simulink model "newthing"  (Simulink 9.1)
settings: Solver=FixedStepAuto  StartTime=0.0  StopTime=tT  FixedStep=dt  RelTol=1e-4  EnableMultiTasking=on
values from neighbouring files (symbols this model uses):
  A = LinearAnalysisToolProject.LocalVariables(2).Value.A    [KalmanFiltBoi.m]    (also in newthingtest.m; newthingtest2.m)
  a1 = 16.235    [LoadQuadrotorConst_XPro1a.m]
  a2 = 17.912    [LoadQuadrotorConst_XPro1a.m]
  a3 = 17.914    [LoadQuadrotorConst_XPro1a.m]
  a4 = 18.161    [LoadQuadrotorConst_XPro1a.m]
  B = LinearAnalysisToolProject.LocalVariables(2).Value.B    [KalmanFiltBoi.m]    (also in newthingtest.m; newthingtest2.m)
  b1 = -0.5036    [LoadQuadrotorConst_XPro1a.m]
  b2 = -12.728    [LoadQuadrotorConst_XPro1a.m]
  b3 = -6.5646    [LoadQuadrotorConst_XPro1a.m]
  b4 = -7.4637    [LoadQuadrotorConst_XPro1a.m]
  c = 0.0002    [LoadQuadrotorConst_XPro1a.m]
  c_mi_x = 170    [LoadQuadrotorConst_XPro1a.m]
  c_mi_y = 170    [LoadQuadrotorConst_XPro1a.m]
  c_mi_z = 40    [LoadQuadrotorConst_XPro1a.m]
  Cc = LinearAnalysisToolProject.LocalVariables(2).Value.C    [newthingtest2.m]
  co_x = 1.7    [LoadQuadrotorConst_XPro1a.m]
  co_y = 1.7    [LoadQuadrotorConst_XPro1a.m]
  co_z = 90.7    [LoadQuadrotorConst_XPro1a.m]
  d = 0.0071    [LoadQuadrotorConst_XPro1a.m]
  d_omega_R10 = 9.1275    [initial_conditions.m]
  d_omega_R20 = 8.955    [initial_conditions.m]
  d_omega_R30 = 8.61    [initial_conditions.m]
  d_omega_R40 = 8.543    [initial_conditions.m]
  dfi_0 = 0    [initial_conditions.m]
  dpsi_0 = 0    [initial_conditions.m]
  dt = 1    [cvx_guidance.m]    (also in newthingtest2.m = 0.01; test_cvx.m = 0.05)
  dtheta_0 = 0    [initial_conditions.m]
  dx_0 = 0    [initial_conditions.m]
  dy_0 = 0    [initial_conditions.m]
  dz_0 = 0    [initial_conditions.m]
  f = 5e-6    (= 5e-06)    [LoadQuadrotorConst_XPro1a.m]
  fi_0 = 0    [initial_conditions.m]
  G = eye(16)    [newthingtest2.m]
  g = 0.0008    [LoadQuadrotorConst_XPro1a.m]    (also in cvx_guidance.m = 9.81)
  ga = 9.807    [LoadQuadrotorConst_XPro1a.m]
  H = eye(16)    [newthingtest2.m]
  h = -0.0282    [LoadQuadrotorConst_XPro1a.m]
  hover = [V1_WP;V2_WP;V3_WP;V4_WP]    [initial_conditions.m]
  Ixx = 2.1385*100    (= 213.85)    [LoadQuadrotorConst_XPro1a.m]
  Iyy = Ixx    (= 213.85)    [LoadQuadrotorConst_XPro1a.m]
  Izz = 3.7479*100    (= 374.79)    [LoadQuadrotorConst_XPro1a.m]
  Jr = 4.86851*0.1    (= 0.486851)    [LoadQuadrotorConst_XPro1a.m]
  K = C(1:4,:)    [newthingtest2.m]
  L = 0.422    [LoadQuadrotorConst_XPro1a.m]
  m = 2.1    [LoadQuadrotorConst_XPro1a.m]    (also in cvx_guidance.m; plot_all_data3D.m = exp(z))
  psi_0 = 0    [initial_conditions.m]
  S_0_0 = 10^7*eye(16)    [newthingtest2.m]
  stateref = [0 0 0 0 0 0 0 0 0 0 0 0 0 0 0 0]'    [newthingtest.m]    (also in newthingtest2.m = [35 0 35 0 50 0 0 0 0 0 0 0 0 0 0 0]')
  Sv = Sv^4    [newthingtest2.m]
  Sw = Sv    [newthingtest2.m]
  Tau = 0.1    [LoadQuadrotorConst_XPro1a.m]
  theta_0 = 0    [initial_conditions.m]
  x_0 = 0    [initial_conditions.m]
  x_0_0 = [x_0 dx_0 y_0 dy_0 z_0 dz_0      fi_0 dfi_0 theta_0 dtheta_0 psi_0 dpsi_0 hover.'].'    [initial_conditions.m]
  y_0 = 0    [initial_conditions.m]
  z_0 = 30    [initial_conditions.m]
settings Model: Creator=Jake  LastModifiedBy=Padraig Lysandrou
settings DataIOCC: LimitDataPoints=on  SignalLoggingSaveFormat=ModelDataLogs
settings OptimizationCC: InitFltsAndDblsToZero=on
settings DebuggingCC: SaveWithParameterizedLinksMsg=none  SignalResolutionControl=TryResolveAllWithWarning  SolverPrmCheckMsg=warning  MultiTaskDSMMsg=warning  MultiTaskCondExecSysMsg=none  FcnCallInpInsideContextMsg=warning
settings SFSimCC: SimParseCustomCode=off
settings GRTTargetCC: TargetFcnLib=ansi_tfl_tmw.mat

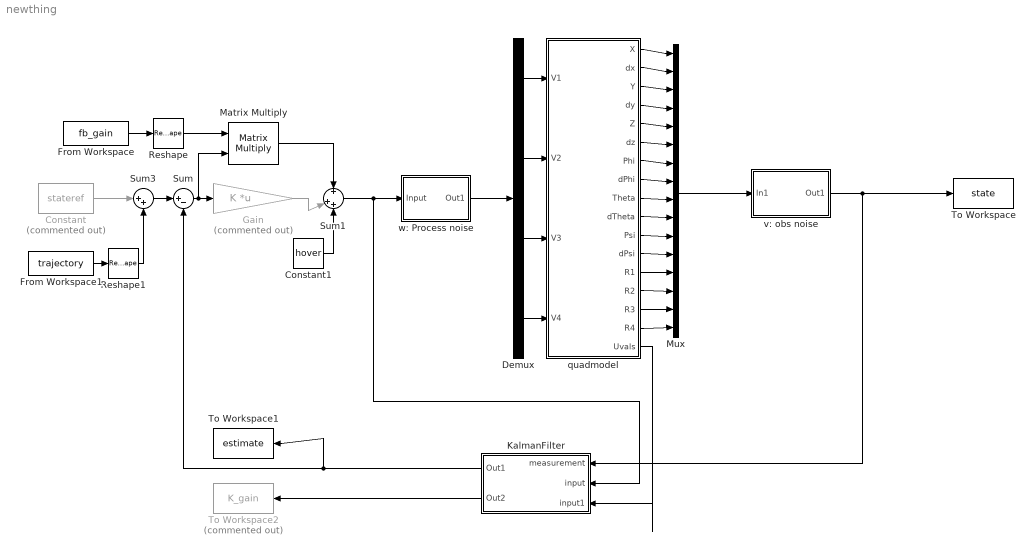
== system newthing ==
  Constant : Constant  Commented=on  Value=stateref
  Constant1 : Constant  Value=hover
  Demux : Demux
  From Workspace : FromWorkspace  VariableName=fb_gain  SampleTime=0
  From Workspace1 : FromWorkspace  VariableName=trajectory  SampleTime=0
  Gain : Gain  Commented=on  Gain=K  Multiplication=Matrix(K*u) (u vector)
  KalmanFilter : Subsystem
  Matrix Multiply : Product  Multiplication=Matrix(*)
  Mux : Mux  Inputs=16
  Reshape : Reshape  OutputDimensionality=Customize  OutputDimensions=[4,16]
  Reshape1 : Reshape  OutputDimensionality=Customize  OutputDimensions=[16,1]
  Sum : Sum  Inputs=|+-
  Sum1 : Sum  Inputs=+|++
  Sum3 : Sum  Inputs=|++
  To Workspace : ToWorkspace  VariableName=state  SaveFormat=Timeseries  SampleTime=-1
  To Workspace1 : ToWorkspace  VariableName=estimate  SaveFormat=Timeseries  SampleTime=-1
  To Workspace2 : ToWorkspace  Commented=on  VariableName=K_gain  SaveFormat=Timeseries  SampleTime=-1
  quadmodel : Subsystem
  v: obs noise : Subsystem
  w: Process noise : Subsystem
  wires:
  quadmodel/1(X) -> Mux/1
  quadmodel/2(dx) -> Mux/2
  quadmodel/3(Y) -> Mux/3
  quadmodel/4(dy) -> Mux/4
  quadmodel/5(Z) -> Mux/5
  quadmodel/6(dz) -> Mux/6
  quadmodel/7(Phi) -> Mux/7
  quadmodel/8(dPhi) -> Mux/8
  quadmodel/9(Theta) -> Mux/9
  quadmodel/10(dTheta) -> Mux/10
  quadmodel/11(Psi) -> Mux/11
  quadmodel/12(dPsi) -> Mux/12
  Demux/1 -> quadmodel/1(V1)
  Demux/2 -> quadmodel/2(V2)
  Demux/3 -> quadmodel/3(V3)
  Demux/4 -> quadmodel/4(V4)
  quadmodel/13(R1) -> Mux/13
  quadmodel/14(R2) -> Mux/14
  quadmodel/15(R3) -> Mux/15
  quadmodel/16(R4) -> Mux/16
  Constant1/1 -> Sum1/3
  From Workspace/1 -> Reshape/1
  Reshape/1 -> Matrix Multiply/1
  Sum/1 -> Matrix Multiply/2, Gain/1
  Matrix Multiply/1 -> Sum1/1
  Gain/1 -> Sum1/2
  From Workspace1/1 -> Reshape1/1
  Sum3/1 -> Sum/1
  Reshape1/1 -> Sum3/2
  Constant/1 -> Sum3/1
  Mux/1 -> v: obs noise/1(In1)
  Sum1/1 -> KalmanFilter/2(input), w: Process noise/1(Input)
  v: obs noise/1(Out1) -> KalmanFilter/1(measurement), To Workspace/1
  w: Process noise/1(Out1) -> Demux/1
  KalmanFilter/2(Out2) -> To Workspace2/1
  KalmanFilter/1(Out1) -> To Workspace1/1, Sum/2
  quadmodel/17(Uvals) -> KalmanFilter/3(input1)

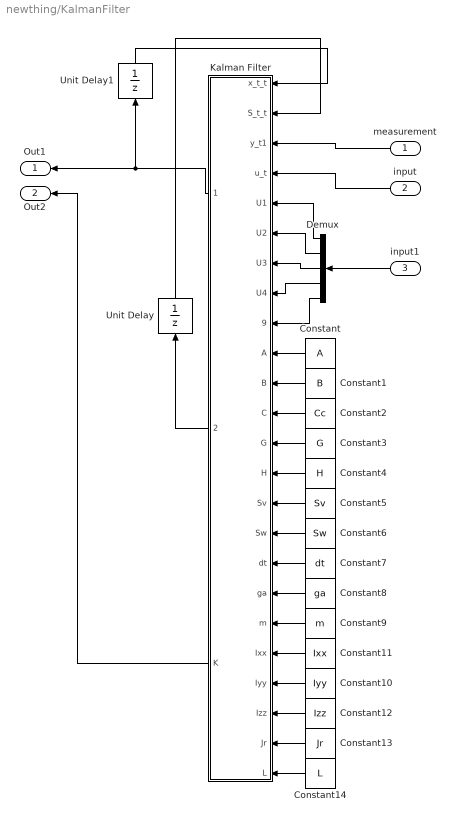
== system newthing/KalmanFilter ==
  measurement : Inport
  input : Inport  Port=2
  input1 : Inport  Port=3
  Constant : Constant  Value=A
  Constant1 : Constant  Value=B
  Constant10 : Constant  Value=Iyy
  Constant11 : Constant  Value=Ixx
  Constant12 : Constant  Value=Izz
  Constant13 : Constant  Value=Jr
  Constant14 : Constant  Value=L
  Constant2 : Constant  Value=Cc
  Constant3 : Constant  Value=G
  Constant4 : Constant  Value=H
  Constant5 : Constant  Value=Sv
  Constant6 : Constant  Value=Sw
  Constant7 : Constant  Value=dt
  Constant8 : Constant  Value=ga
  Constant9 : Constant  Value=m
  Demux : Demux  Outputs=5
  Kalman Filter : MATLAB Function  TreatAsAtomicUnit=on
  Unit Delay : UnitDelay  InitialCondition=S_0_0  SampleTime=-1
  Unit Delay1 : UnitDelay  InitialCondition=x_0_0  SampleTime=-1
  Out1 : Outport
  Out2 : Outport  Port=2
  wires:
  Kalman Filter/1(x_t1_t1) -> Unit Delay1/1, Out1/1
  Constant/1 -> Kalman Filter/10(A)
  Constant1/1 -> Kalman Filter/11(B)
  Constant2/1 -> Kalman Filter/12(C)
  Kalman Filter/2(S_t1_t1) -> Unit Delay/1
  Unit Delay/1 -> Kalman Filter/2(S_t_t)
  Unit Delay1/1 -> Kalman Filter/1(x_t_t)
  Constant3/1 -> Kalman Filter/13(G)
  Constant4/1 -> Kalman Filter/14(H)
  Constant5/1 -> Kalman Filter/15(Sv)
  Constant6/1 -> Kalman Filter/16(Sw)
  Kalman Filter/3(K) -> Out2/1
  measurement/1 -> Kalman Filter/3(y_t1)
  Demux/1 -> Kalman Filter/5(U1)
  Demux/2 -> Kalman Filter/6(U2)
  Demux/3 -> Kalman Filter/7(U3)
  Demux/4 -> Kalman Filter/8(U4)
  Demux/5 -> Kalman Filter/9(Omega)
  input1/1 -> Demux/1
  input/1 -> Kalman Filter/4(u_t)
  Constant7/1 -> Kalman Filter/17(dt)
  Constant8/1 -> Kalman Filter/18(ga)
  Constant9/1 -> Kalman Filter/19(m)
  Constant10/1 -> Kalman Filter/21(Iyy)
  Constant11/1 -> Kalman Filter/20(Ixx)
  Constant12/1 -> Kalman Filter/22(Izz)
  Constant14/1 -> Kalman Filter/24(L)
  Constant13/1 -> Kalman Filter/23(Jr)

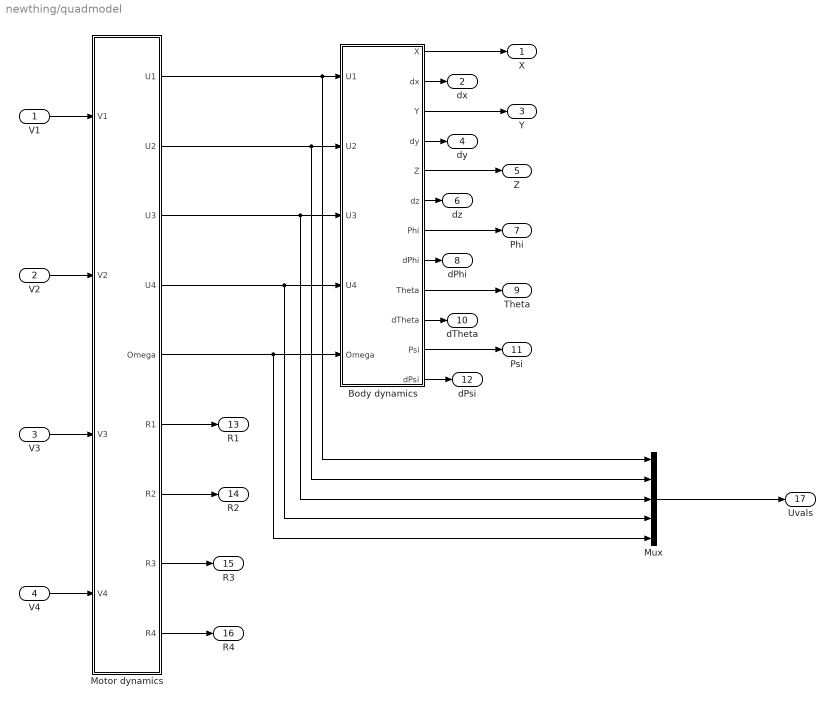
== system newthing/quadmodel ==
  V1 : Inport
  V2 : Inport  Port=2
  V3 : Inport  Port=3
  V4 : Inport  Port=4
  Body dynamics : Subsystem
  Motor dynamics : Subsystem
  Mux : Mux  Inputs=5
  X : Outport
  dx : Outport  Port=2
  Y : Outport  Port=3
  dy : Outport  Port=4
  Z : Outport  Port=5
  dz : Outport  Port=6
  Phi : Outport  Port=7
  dPhi : Outport  Port=8
  Theta : Outport  Port=9
  dTheta : Outport  Port=10
  Psi : Outport  Port=11
  dPsi : Outport  Port=12
  R1 : Outport  Port=13
  R2 : Outport  Port=14
  R3 : Outport  Port=15
  R4 : Outport  Port=16
  Uvals : Outport  Port=17
  wires:
  Motor dynamics/1(U1) -> Body dynamics/1(U1), Mux/1
  Motor dynamics/2(U2) -> Body dynamics/2(U2), Mux/2
  Motor dynamics/3(U3) -> Body dynamics/3(U3), Mux/3
  Motor dynamics/4(U4) -> Body dynamics/4(U4), Mux/4
  Motor dynamics/5(Omega) -> Body dynamics/5(Omega), Mux/5
  Body dynamics/7(Phi) -> Phi/1
  Body dynamics/9(Theta) -> Theta/1
  Body dynamics/11(Psi) -> Psi/1
  Body dynamics/1(X) -> X/1
  V1/1 -> Motor dynamics/1(V1)
  Body dynamics/3(Y) -> Y/1
  V2/1 -> Motor dynamics/2(V2)
  Body dynamics/5(Z) -> Z/1
  V3/1 -> Motor dynamics/3(V3)
  V4/1 -> Motor dynamics/4(V4)
  Body dynamics/2(dx) -> dx/1
  Body dynamics/4(dy) -> dy/1
  Body dynamics/6(dz) -> dz/1
  Body dynamics/8(dPhi) -> dPhi/1
  Body dynamics/10(dTheta) -> dTheta/1
  Body dynamics/12(dPsi) -> dPsi/1
  Motor dynamics/6(R1) -> R1/1
  Motor dynamics/7(R2) -> R2/1
  Motor dynamics/8(R3) -> R3/1
  Motor dynamics/9(R4) -> R4/1
  Mux/1 -> Uvals/1

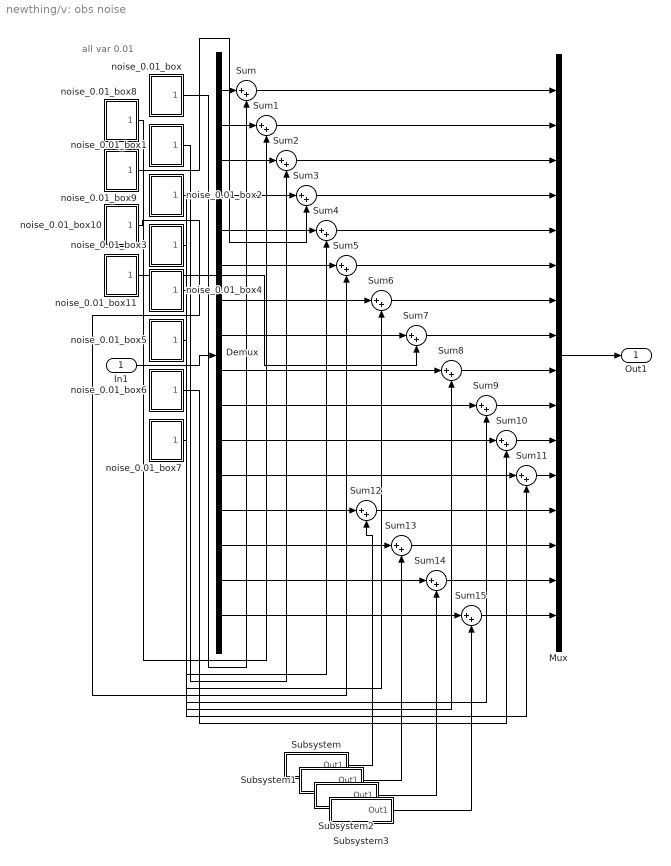
== system newthing/v: obs noise ==
  note: all var 0.01
  In1 : Inport
  Demux : Demux  Outputs=16
  Mux : Mux  Inputs=16
  Subsystem : Subsystem
  Subsystem1 : Subsystem
  Subsystem2 : Subsystem
  Subsystem3 : Subsystem
  Sum{,1..15} (16 alike) : Sum  Inputs=|++
  noise_0.01_box : Subsystem
  noise_0.01_box1 : Subsystem
  noise_0.01_box10 : Subsystem
  noise_0.01_box11 : Subsystem
  noise_0.01_box2 : Subsystem
  noise_0.01_box3 : Subsystem
  noise_0.01_box4 : Subsystem
  noise_0.01_box5 : Subsystem
  noise_0.01_box6 : Subsystem
  noise_0.01_box7 : Subsystem
  noise_0.01_box8 : Subsystem
  noise_0.01_box9 : Subsystem
  Out1 : Outport
  wires:
  Demux/2 -> Sum1/1
  Demux/1 -> Sum/1
  Sum2/1 -> Mux/3
  Sum/1 -> Mux/1
  Demux/3 -> Sum2/1
  Demux/4 -> Sum3/1
  Sum3/1 -> Mux/4
  Demux/5 -> Sum4/1
  Sum4/1 -> Mux/5
  Sum1/1 -> Mux/2
  Demux/6 -> Sum5/1
  Sum5/1 -> Mux/6
  Demux/7 -> Sum6/1
  Sum6/1 -> Mux/7
  Demux/8 -> Sum7/1
  Sum7/1 -> Mux/8
  Demux/9 -> Sum8/1
  Sum8/1 -> Mux/9
  Demux/10 -> Sum9/1
  Sum9/1 -> Mux/10
  Demux/11 -> Sum10/1
  Sum10/1 -> Mux/11
  Demux/12 -> Sum11/1
  Sum11/1 -> Mux/12
  In1/1 -> Demux/1
  Mux/1 -> Out1/1
  Demux/13 -> Sum12/1
  Sum12/1 -> Mux/13
  Demux/14 -> Sum13/1
  Sum13/1 -> Mux/14
  Demux/15 -> Sum14/1
  Sum14/1 -> Mux/15
  Demux/16 -> Sum15/1
  Sum15/1 -> Mux/16
  noise_0.01_box/1(Out1) -> Sum/2
  noise_0.01_box8/1(Out1) -> Sum1/2
  noise_0.01_box1/1(Out1) -> Sum2/2
  noise_0.01_box9/1(Out1) -> Sum3/2
  noise_0.01_box2/1(Out1) -> Sum4/2
  noise_0.01_box10/1(Out1) -> Sum5/2
  noise_0.01_box3/1(Out1) -> Sum6/2
  noise_0.01_box11/1(Out1) -> Sum7/2
  noise_0.01_box4/1(Out1) -> Sum8/2
  noise_0.01_box5/1(Out1) -> Sum9/2
  noise_0.01_box6/1(Out1) -> Sum10/2
  noise_0.01_box7/1(Out1) -> Sum11/2
  Subsystem/1(Out1) -> Sum12/2
  Subsystem1/1(Out1) -> Sum13/2
  Subsystem2/1(Out1) -> Sum14/2
  Subsystem3/1(Out1) -> Sum15/2

== system newthing/w: Process noise ==
  Input : Inport
  Demux : Demux
  Mux : Mux
  Subsystem : Subsystem
  Subsystem1 : Subsystem
  Subsystem2 : Subsystem
  Subsystem3 : Subsystem
  Sum{,1..3} (4 alike) : Sum  Inputs=|++
  Out1 : Outport
  wires:
  Input/1 -> Demux/1
  Demux/1 -> Sum/1
  Demux/2 -> Sum1/1
  Mux/1 -> Out1/1
  Sum/1 -> Mux/1
  Sum1/1 -> Mux/2
  Demux/3 -> Sum2/1
  Demux/4 -> Sum3/1
  Sum2/1 -> Mux/3
  Sum3/1 -> Mux/4
  Subsystem/1(Out1) -> Sum3/2
  Subsystem1/1(Out1) -> Sum2/2
  Subsystem2/1(Out1) -> Sum1/2
  Subsystem3/1(Out1) -> Sum/2

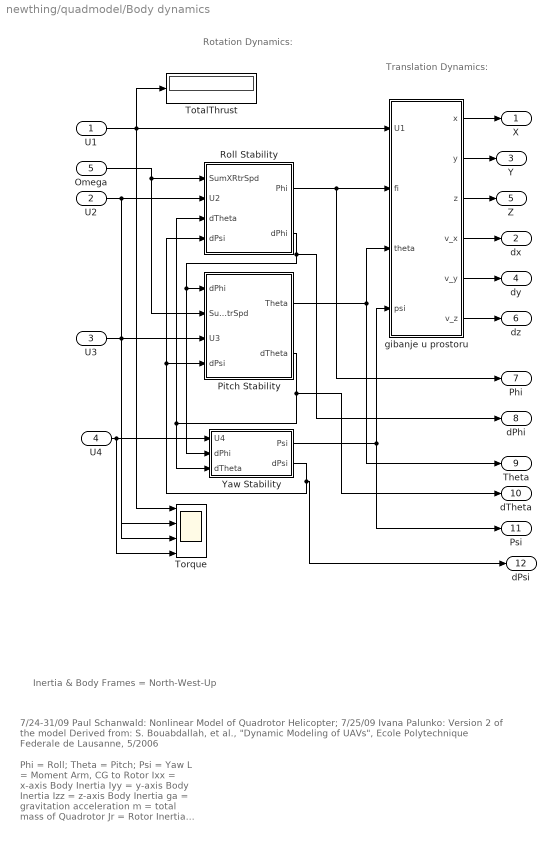
== system newthing/quadmodel/Body dynamics ==
  note: Inertia & Body Frames = North-West-Up
  note: Rotation
      | Dynamics:
  note: Translation
      | Dynamics:
  note: Phi = Roll; Theta = Pitch; Psi = Yaw
      | L = Moment Arm, CG to Rotor
      | Ixx = x-axis Body Inertia
      | Iyy = y-axis Body Inertia
      | Izz = z-axis Body Inertia
      | ga = gravitation acceleration
      | m = total mass of Quadrotor
      | Jr = Rotor Inertia
      | a,b = Volts-to-Rotor Speed Consts
      | c,d,e = RtrSpd-to-Thrust Fcn Consts
      | f,g,h = RtrSpd-to-Drag Fcn Consts
      | Tau = Motor Time Const
  note: 7/24-31/09  Paul Schanwald:  Nonlinear Model of Quadrotor Helicopter; 7/25/09 Ivana Palunko: Version 2 of the model
      | Derived from: S. Bouabdallah, et al., "Dynamic Modeling of UAVs", Ecole Polytechnique Federale de Lausanne, 5/2006
  U1 : Inport
  U2 : Inport  Port=2
  U3 : Inport  Port=3
  U4 : Inport  Port=4
  Omega : Inport  Port=5
  Pitch Stability : Subsystem
  Roll Stability : Subsystem
  Torque : Scope  NumInputPorts=4
  TotalThrust : Display
  Yaw Stability : Subsystem
  gibanje u prostoru : Subsystem
  X : Outport
  dx : Outport  Port=2
  Y : Outport  Port=3
  dy : Outport  Port=4
  Z : Outport  Port=5
  dz : Outport  Port=6
  Phi : Outport  Port=7
  dPhi : Outport  Port=8
  Theta : Outport  Port=9
  dTheta : Outport  Port=10
  Psi : Outport  Port=11
  dPsi : Outport  Port=12
  wires:
  U4/1 -> Yaw Stability/1(U4), Torque/4
  U3/1 -> Pitch Stability/3(U3), Torque/3
  U1/1 -> TotalThrust/1, gibanje u prostoru/1(U1), Torque/1
  gibanje u prostoru/3(z) -> Z/1
  gibanje u prostoru/2(y) -> Y/1
  gibanje u prostoru/1(x) -> X/1
  U2/1 -> Roll Stability/2(U2), Torque/2
  Omega/1 -> Roll Stability/1(SumXRtrSpd), Pitch Stability/2(SumYRtrSpd)
  Roll Stability/2(dPhi) -> dPhi/1, Pitch Stability/1(dPhi), Yaw Stability/2(dPhi)
  Pitch Stability/2(dTheta) -> dTheta/1, Yaw Stability/3(dTheta), Roll Stability/3(dTheta)
  Yaw Stability/2(dPsi) -> dPsi/1, Roll Stability/4(dPsi), Pitch Stability/4(dPsi)
  Roll Stability/1(Phi) -> gibanje u prostoru/2(fi), Phi/1
  Pitch Stability/1(Theta) -> gibanje u prostoru/3(theta), Theta/1
  Yaw Stability/1(Psi) -> Psi/1, gibanje u prostoru/4(psi)
  gibanje u prostoru/6(v_z) -> dz/1
  gibanje u prostoru/4(v_x) -> dx/1
  gibanje u prostoru/5(v_y) -> dy/1

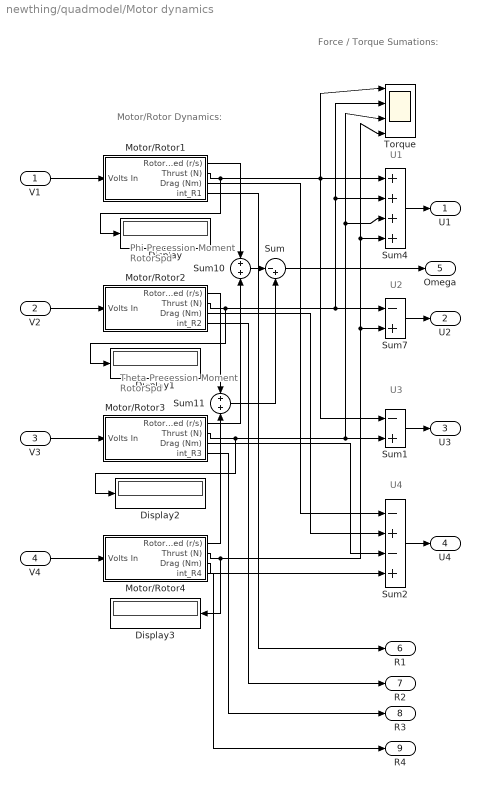
== system newthing/quadmodel/Motor dynamics ==
  note: Theta Precession
      | Moment RotorSpd
  note: Phi Precession
      | Moment RotorSpd
  note: Motor/Rotor
      | Dynamics:
  note: Force / Torque
      | Sumations:
  note: U4
  note: U3
  note: U2
  note: U1
  V1 : Inport
  V2 : Inport  Port=2
  V3 : Inport  Port=3
  V4 : Inport  Port=4
  Display{,1..3} (4 alike) : Display
  Motor/Rotor1 : Subsystem
  Motor/Rotor2 : Subsystem
  Motor/Rotor3 : Subsystem
  Motor/Rotor4 : Subsystem
  Sum : Sum  Inputs=|-+
  Sum1 : Sum  Inputs=-+
  Sum10 : Sum  Inputs=+|+
  Sum11 : Sum  Inputs=+|+
  Sum2 : Sum  Inputs=-+-+
  Sum4 : Sum  Inputs=++++
  Sum7 : Sum  Inputs=-+
  Torque : Scope  NumInputPorts=4
  U1 : Outport
  U2 : Outport  Port=2
  U3 : Outport  Port=3
  U4 : Outport  Port=4
  Omega : Outport  Port=5
  R1 : Outport  Port=6
  R2 : Outport  Port=7
  R3 : Outport  Port=8
  R4 : Outport  Port=9
  wires:
  Sum11/1 -> Sum/2
  Sum10/1 -> Sum/1
  Motor/Rotor4/1(Rotor Speed (r/s)) -> Sum11/2
  Motor/Rotor4/2(Thrust (N)) -> Display3/1, Torque/4, Sum4/4, Sum7/2
  Motor/Rotor4/3(Drag (Nm)) -> Sum2/4
  Motor/Rotor3/3(Drag (Nm)) -> Sum2/3
  Motor/Rotor3/1(Rotor Speed (r/s)) -> Sum10/2
  Motor/Rotor3/2(Thrust (N)) -> Display2/1, Torque/3, Sum4/3, Sum1/2
  Motor/Rotor2/1(Rotor Speed (r/s)) -> Sum11/1
  Motor/Rotor2/3(Drag (Nm)) -> Sum2/2
  Motor/Rotor2/2(Thrust (N)) -> Display1/1, Torque/2, Sum4/2, Sum7/1
  Motor/Rotor1/1(Rotor Speed (r/s)) -> Sum10/1
  Motor/Rotor1/3(Drag (Nm)) -> Sum2/1
  Motor/Rotor1/2(Thrust (N)) -> Display/1, Sum4/1, Torque/1, Sum1/1
  Sum4/1 -> U1/1
  Sum/1 -> Omega/1
  Sum7/1 -> U2/1
  Sum1/1 -> U3/1
  Sum2/1 -> U4/1
  V1/1 -> Motor/Rotor1/1(Volts In)
  V2/1 -> Motor/Rotor2/1(Volts In)
  V3/1 -> Motor/Rotor3/1(Volts In)
  V4/1 -> Motor/Rotor4/1(Volts In)
  Motor/Rotor1/4(int_R1) -> R1/1
  Motor/Rotor2/4(int_R2) -> R2/1
  Motor/Rotor3/4(int_R3) -> R3/1
  Motor/Rotor4/4(int_R4) -> R4/1

== system newthing/v: obs noise/Subsystem ==
  Constant1 : Constant  Value=0.0001
  Multiply1 : Product
  Random Number1 : RandomNumber  Variance=0.0001  SampleTime=dt
  Out1 : Outport
  wires:
  Multiply1/1 -> Out1/1
  Random Number1/1 -> Multiply1/2
  Constant1/1 -> Multiply1/1

== system newthing/v: obs noise/Subsystem1 ==
  Constant1 : Constant  Value=0.0001
  Multiply1 : Product
  Random Number1 : RandomNumber  Variance=0.0001  SampleTime=dt
  Out1 : Outport
  wires:
  Multiply1/1 -> Out1/1
  Random Number1/1 -> Multiply1/2
  Constant1/1 -> Multiply1/1

== system newthing/v: obs noise/Subsystem2 ==
  Constant1 : Constant  Value=0.0001
  Multiply1 : Product
  Random Number1 : RandomNumber  Variance=0.0001  SampleTime=dt
  Out1 : Outport
  wires:
  Multiply1/1 -> Out1/1
  Random Number1/1 -> Multiply1/2
  Constant1/1 -> Multiply1/1

== system newthing/v: obs noise/Subsystem3 ==
  Constant1 : Constant  Value=0.0001
  Multiply1 : Product
  Random Number1 : RandomNumber  Variance=0.0001  SampleTime=dt
  Out1 : Outport
  wires:
  Multiply1/1 -> Out1/1
  Random Number1/1 -> Multiply1/2
  Constant1/1 -> Multiply1/1

== system newthing/v: obs noise/noise_0.01_box ==
  Constant2 : Constant  Value=0.01
  Multiply : Product
  Random Number : RandomNumber  Variance=0.01  SampleTime=dt
  Out1 : Outport
  wires:
  Random Number/1 -> Multiply/2
  Constant2/1 -> Multiply/1
  Multiply/1 -> Out1/1

== system newthing/v: obs noise/noise_0.01_box1 ==
  Constant2 : Constant  Value=0.01
  Multiply : Product
  Random Number : RandomNumber  Variance=0.01  SampleTime=dt
  Out1 : Outport
  wires:
  Random Number/1 -> Multiply/2
  Constant2/1 -> Multiply/1
  Multiply/1 -> Out1/1

== system newthing/v: obs noise/noise_0.01_box10 ==
  Constant2 : Constant  Value=0.01
  Multiply : Product
  Random Number : RandomNumber  Variance=0.01  SampleTime=dt
  Out1 : Outport
  wires:
  Random Number/1 -> Multiply/2
  Constant2/1 -> Multiply/1
  Multiply/1 -> Out1/1

== system newthing/v: obs noise/noise_0.01_box11 ==
  Constant2 : Constant  Value=0.01
  Multiply : Product
  Random Number : RandomNumber  Variance=0.01  SampleTime=dt
  Out1 : Outport
  wires:
  Random Number/1 -> Multiply/2
  Constant2/1 -> Multiply/1
  Multiply/1 -> Out1/1

== system newthing/v: obs noise/noise_0.01_box2 ==
  Constant2 : Constant  Value=0.01
  Multiply : Product
  Random Number : RandomNumber  Variance=0.01  SampleTime=dt
  Out1 : Outport
  wires:
  Random Number/1 -> Multiply/2
  Constant2/1 -> Multiply/1
  Multiply/1 -> Out1/1

== system newthing/v: obs noise/noise_0.01_box3 ==
  Constant2 : Constant  Value=0.01
  Multiply : Product
  Random Number : RandomNumber  Variance=0.01  SampleTime=dt
  Out1 : Outport
  wires:
  Random Number/1 -> Multiply/2
  Constant2/1 -> Multiply/1
  Multiply/1 -> Out1/1

== system newthing/v: obs noise/noise_0.01_box4 ==
  Constant2 : Constant  Value=0.01
  Multiply : Product
  Random Number : RandomNumber  Variance=0.01  SampleTime=dt
  Out1 : Outport
  wires:
  Random Number/1 -> Multiply/2
  Constant2/1 -> Multiply/1
  Multiply/1 -> Out1/1

== system newthing/v: obs noise/noise_0.01_box5 ==
  Constant2 : Constant  Value=0.01
  Multiply : Product
  Random Number : RandomNumber  Variance=0.01  SampleTime=dt
  Out1 : Outport
  wires:
  Random Number/1 -> Multiply/2
  Constant2/1 -> Multiply/1
  Multiply/1 -> Out1/1

== system newthing/v: obs noise/noise_0.01_box6 ==
  Constant2 : Constant  Value=0.01
  Multiply : Product
  Random Number : RandomNumber  Variance=0.01  SampleTime=dt
  Out1 : Outport
  wires:
  Random Number/1 -> Multiply/2
  Constant2/1 -> Multiply/1
  Multiply/1 -> Out1/1

== system newthing/v: obs noise/noise_0.01_box7 ==
  Constant2 : Constant  Value=0.01
  Multiply : Product
  Random Number : RandomNumber  Variance=0.01  SampleTime=dt
  Out1 : Outport
  wires:
  Random Number/1 -> Multiply/2
  Constant2/1 -> Multiply/1
  Multiply/1 -> Out1/1

== system newthing/v: obs noise/noise_0.01_box8 ==
  Constant2 : Constant  Value=0.01
  Multiply : Product
  Random Number : RandomNumber  Variance=0.01  SampleTime=dt
  Out1 : Outport
  wires:
  Random Number/1 -> Multiply/2
  Constant2/1 -> Multiply/1
  Multiply/1 -> Out1/1

== system newthing/v: obs noise/noise_0.01_box9 ==
  Constant2 : Constant  Value=0.01
  Multiply : Product
  Random Number : RandomNumber  Variance=0.01  SampleTime=dt
  Out1 : Outport
  wires:
  Random Number/1 -> Multiply/2
  Constant2/1 -> Multiply/1
  Multiply/1 -> Out1/1

== system newthing/w: Process noise/Subsystem ==
  Constant2 : Constant  Value=0.05
  Multiply : Product
  Random Number : RandomNumber  Variance=0.05  SampleTime=dt
  Out1 : Outport
  wires:
  Multiply/1 -> Out1/1
  Random Number/1 -> Multiply/2
  Constant2/1 -> Multiply/1

== system newthing/w: Process noise/Subsystem1 ==
  Constant2 : Constant  Value=0.05
  Multiply : Product
  Random Number : RandomNumber  Variance=0.05  SampleTime=dt
  Out1 : Outport
  wires:
  Multiply/1 -> Out1/1
  Random Number/1 -> Multiply/2
  Constant2/1 -> Multiply/1

== system newthing/w: Process noise/Subsystem2 ==
  Constant2 : Constant  Value=0.05
  Multiply : Product
  Random Number : RandomNumber  Variance=0.05  SampleTime=dt
  Out1 : Outport
  wires:
  Multiply/1 -> Out1/1
  Random Number/1 -> Multiply/2
  Constant2/1 -> Multiply/1

== system newthing/w: Process noise/Subsystem3 ==
  Constant2 : Constant  Value=0.05
  Multiply : Product
  Random Number : RandomNumber  Variance=0.05  SampleTime=dt
  Out1 : Outport
  wires:
  Multiply/1 -> Out1/1
  Random Number/1 -> Multiply/2
  Constant2/1 -> Multiply/1

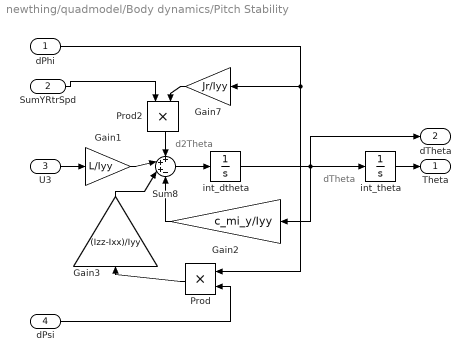
== system newthing/quadmodel/Body dynamics/Pitch Stability ==
  note: d2Theta
  note: dTheta
  dPhi : Inport
  SumYRtrSpd : Inport  Port=2
  U3 : Inport  Port=3
  dPsi : Inport  Port=4
  Gain1 : Gain  Gain=L/Iyy
  Gain2 : Gain  Gain=c_mi_y/Iyy
  Gain3 : Gain  Gain=(Izz-Ixx)/Iyy
  Gain7 : Gain  Gain=Jr/Iyy
  Prod : Product  RndMeth=Zero
  Prod2 : Product  RndMeth=Zero
  Sum8 : Sum  Inputs=+++-
  int_dtheta : Integrator  InitialCondition=dtheta_0
  int_theta : Integrator  InitialCondition=theta_0  UpperSaturationLimit=pi/2  LowerSaturationLimit=-pi/2
  Theta : Outport
  dTheta : Outport  Port=2
  wires:
  Gain2/1 -> Sum8/4
  dPhi/1 -> Prod/1, Gain7/1
  int_theta/1 -> Theta/1
  U3/1 -> Gain1/1
  SumYRtrSpd/1 -> Prod2/1
  dPsi/1 -> Prod/2
  int_dtheta/1 -> dTheta/1, int_theta/1, Gain2/1
  Sum8/1 -> int_dtheta/1
  Gain1/1 -> Sum8/2
  Gain7/1 -> Prod2/2
  Gain3/1 -> Sum8/3
  Prod/1 -> Gain3/1
  Prod2/1 -> Sum8/1

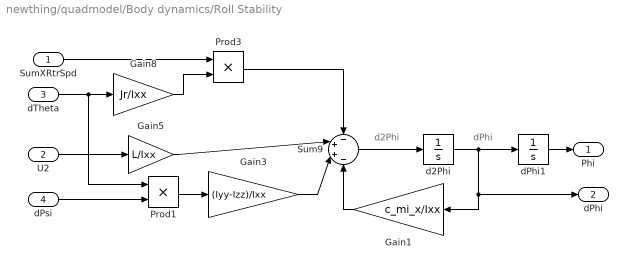
== system newthing/quadmodel/Body dynamics/Roll Stability ==
  note: d2Phi
  note: dPhi
  SumXRtrSpd : Inport
  U2 : Inport  Port=2
  dTheta : Inport  Port=3
  dPsi : Inport  Port=4
  Gain1 : Gain  Gain=c_mi_x/Ixx
  Gain3 : Gain  Gain=(Iyy-Izz)/Ixx
  Gain5 : Gain  Gain=L/Ixx
  Gain8 : Gain  Gain=Jr/Ixx
  Prod1 : Product  RndMeth=Zero
  Prod3 : Product  RndMeth=Zero
  Sum9 : Sum  Inputs=-++-
  d2Phi : Integrator  InitialCondition=dfi_0
  dPhi1 : Integrator  InitialCondition=fi_0  UpperSaturationLimit=pi/2  LowerSaturationLimit=-pi/2
  Phi : Outport
  dPhi : Outport  Port=2
  wires:
  dPsi/1 -> Prod1/2
  dTheta/1 -> Prod1/1, Gain8/1
  Prod3/1 -> Sum9/1
  SumXRtrSpd/1 -> Prod3/1
  Gain8/1 -> Prod3/2
  dPhi1/1 -> Phi/1
  U2/1 -> Gain5/1
  d2Phi/1 -> Gain1/1, dPhi/1, dPhi1/1
  Sum9/1 -> d2Phi/1
  Gain5/1 -> Sum9/2
  Gain1/1 -> Sum9/4
  Gain3/1 -> Sum9/3
  Prod1/1 -> Gain3/1

== system newthing/quadmodel/Body dynamics/Yaw Stability ==
  note: dPsi
  note: d2Psi
  U4 : Inport
  dPhi : Inport  Port=2
  dTheta : Inport  Port=3
  Gain : Gain  Gain=1/Izz
  Gain1 : Gain  Gain=c_mi_z
  Gain2 : Gain  Gain=Ixx-Iyy
  Product : Product  RndMeth=Zero
  Sum : Sum  Inputs=|++-
  ind_dpsi : Integrator  InitialCondition=dpsi_0
  int_psi : Integrator  InitialCondition=psi_0
  Psi : Outport
  dPsi : Outport  Port=2
  wires:
  Sum/1 -> Gain/1
  U4/1 -> Sum/1
  int_psi/1 -> Psi/1
  Gain/1 -> ind_dpsi/1
  ind_dpsi/1 -> Gain1/1, dPsi/1, int_psi/1
  Gain1/1 -> Sum/3
  Gain2/1 -> Sum/2
  dPhi/1 -> Product/1
  dTheta/1 -> Product/2
  Product/1 -> Gain2/1

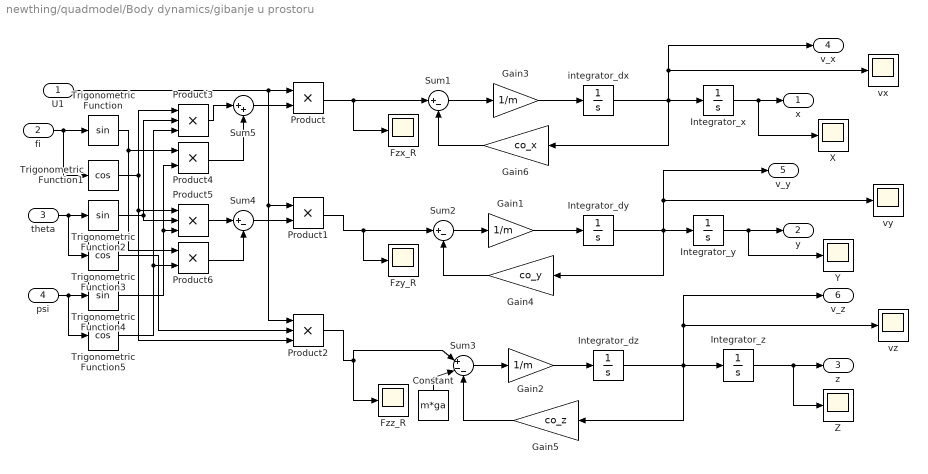
== system newthing/quadmodel/Body dynamics/gibanje u prostoru ==
  U1 : Inport
  fi : Inport  Port=2
  theta : Inport  Port=3
  psi : Inport  Port=4
  Constant : Constant  Value=m*ga
  Fzx_R : Scope
  Fzy_R : Scope
  Fzz_R : Scope
  Gain1 : Gain  Gain=1/m
  Gain2 : Gain  Gain=1/m
  Gain3 : Gain  Gain=1/m
  Gain4 : Gain  Gain=co_y
  Gain5 : Gain  Gain=co_z
  Gain6 : Gain  Gain=co_x
  Integrator_dy : Integrator  InitialCondition=dy_0  LimitOutput=on  UpperSaturationLimit=10  LowerSaturationLimit=-10
  Integrator_dz : Integrator  InitialCondition=dz_0  LimitOutput=on  UpperSaturationLimit=10  LowerSaturationLimit=-10
  Integrator_x : Integrator  InitialCondition=x_0
  Integrator_y : Integrator  InitialCondition=y_0
  Integrator_z : Integrator  InitialCondition=z_0
  Product{,1,4,6} (4 alike) : Product  RndMeth=Zero
  Product2 : Product  Inputs=3  RndMeth=Zero
  Product3 : Product  Inputs=3  RndMeth=Zero
  Product5 : Product  Inputs=3  RndMeth=Zero
  Sum1 : Sum  Inputs=|+-
  Sum2 : Sum  Inputs=|+-
  Sum3 : Sum  Inputs=|+--
  Sum4 : Sum  Inputs=|+-
  Sum5 : Sum  Inputs=|++
  Trigonometric Function : Trigonometry
  Trigonometric Function1 : Trigonometry  Operator=cos
  Trigonometric Function2 : Trigonometry
  Trigonometric Function3 : Trigonometry  Operator=cos
  Trigonometric Function4 : Trigonometry
  Trigonometric Function5 : Trigonometry  Operator=cos
  X : Scope
  Y : Scope
  Z : Scope
  integrator_dx : Integrator  InitialCondition=dx_0  LimitOutput=on  UpperSaturationLimit=10  LowerSaturationLimit=-10
  vx : Scope
  vy : Scope
  vz : Scope
  x : Outport
  y : Outport  Port=2
  z : Outport  Port=3
  v_x : Outport  Port=4
  v_y : Outport  Port=5
  v_z : Outport  Port=6
  wires:
  Gain5/1 -> Sum3/3
  Constant/1 -> Sum3/2
  Gain4/1 -> Sum2/2
  Sum3/1 -> Gain2/1
  Gain6/1 -> Sum1/2
  Product2/1 -> Sum3/1, Fzz_R/1
  Sum2/1 -> Gain1/1
  Product1/1 -> Fzy_R/1, Sum2/1
  Gain2/1 -> Integrator_dz/1
  Sum1/1 -> Gain3/1
  Product/1 -> Fzx_R/1, Sum1/1
  U1/1 -> Product/1, Product1/1, Product2/1
  Integrator_y/1 -> Y/1, y/1
  Integrator_x/1 -> X/1, x/1
  Integrator_z/1 -> Z/1, z/1
  integrator_dx/1 -> Gain6/1, vx/1, v_x/1, Integrator_x/1
  Integrator_dy/1 -> Gain4/1, Integrator_y/1, vy/1, v_y/1
  Integrator_dz/1 -> vz/1, v_z/1, Gain5/1, Integrator_z/1
  Gain1/1 -> Integrator_dy/1
  Gain3/1 -> integrator_dx/1
  Sum4/1 -> Product1/2
  Sum5/1 -> Product/2
  Product3/1 -> Sum5/1
  Product4/1 -> Sum5/2
  Product5/1 -> Sum4/1
  Product6/1 -> Sum4/2
  psi/1 -> Trigonometric Function4/1, Trigonometric Function5/1
  theta/1 -> Trigonometric Function2/1, Trigonometric Function3/1
  fi/1 -> Trigonometric Function/1, Trigonometric Function1/1
  Trigonometric Function/1 -> Product4/1, Product6/1
  Trigonometric Function1/1 -> Product3/1, Product5/1, Product2/3
  Trigonometric Function2/1 -> Product3/2, Product5/2
  Trigonometric Function5/1 -> Product3/3, Product6/2
  Trigonometric Function4/1 -> Product4/2, Product5/3
  Trigonometric Function3/1 -> Product2/2

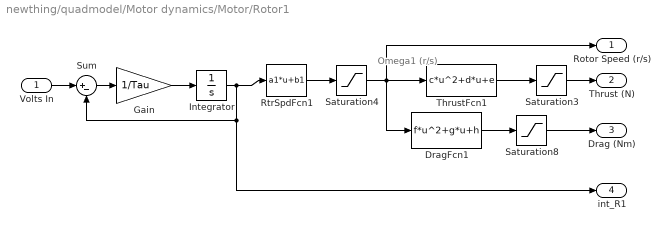
== system newthing/quadmodel/Motor dynamics/Motor/Rotor1 ==
  note: Omega1
      | (r/s)
  Volts In : Inport
  DragFcn1 : Fcn  Expr=f*u^2+g*u+h
  Gain : Gain  Gain=1/Tau
  Integrator : Integrator  InitialCondition=d_omega_R10
  RtrSpdFcn1 : Fcn  Expr=a1*u+b1
  Saturation3 : Saturate  UpperLimit=15  LowerLimit=0
  Saturation4 : Saturate  UpperLimit=250  LowerLimit=0
  Saturation8 : Saturate  UpperLimit=1  LowerLimit=0
  Sum : Sum  Inputs=|+-
  ThrustFcn1 : Fcn  Expr=c*u^2+d*u+e
  Rotor Speed (r/s) : Outport
  Thrust (N) : Outport  Port=2
  Drag (Nm) : Outport  Port=3
  int_R1 : Outport  Port=4
  wires:
  Volts In/1 -> Sum/1
  Sum/1 -> Gain/1
  Integrator/1 -> RtrSpdFcn1/1, int_R1/1, Sum/2
  Gain/1 -> Integrator/1
  Saturation3/1 -> Thrust (N)/1
  Saturation8/1 -> Drag (Nm)/1
  DragFcn1/1 -> Saturation8/1
  Saturation4/1 -> Rotor Speed (r/s)/1, DragFcn1/1, ThrustFcn1/1
  RtrSpdFcn1/1 -> Saturation4/1
  ThrustFcn1/1 -> Saturation3/1

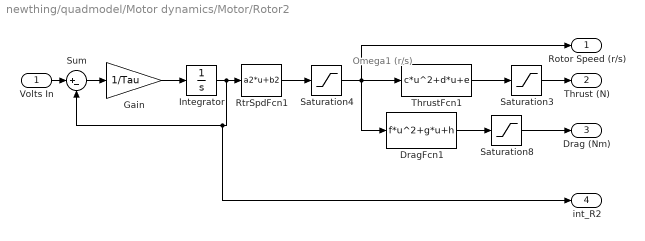
== system newthing/quadmodel/Motor dynamics/Motor/Rotor2 ==
  note: Omega1
      | (r/s)
  Volts In : Inport
  DragFcn1 : Fcn  Expr=f*u^2+g*u+h
  Gain : Gain  Gain=1/Tau
  Integrator : Integrator  InitialCondition=d_omega_R20
  RtrSpdFcn1 : Fcn  Expr=a2*u+b2
  Saturation3 : Saturate  UpperLimit=15  LowerLimit=0
  Saturation4 : Saturate  UpperLimit=250  LowerLimit=0
  Saturation8 : Saturate  UpperLimit=1  LowerLimit=0
  Sum : Sum  Inputs=|+-
  ThrustFcn1 : Fcn  Expr=c*u^2+d*u+e
  Rotor Speed (r/s) : Outport
  Thrust (N) : Outport  Port=2
  Drag (Nm) : Outport  Port=3
  int_R2 : Outport  Port=4
  wires:
  Volts In/1 -> Sum/1
  Sum/1 -> Gain/1
  Integrator/1 -> RtrSpdFcn1/1, int_R2/1, Sum/2
  Gain/1 -> Integrator/1
  Saturation3/1 -> Thrust (N)/1
  Saturation8/1 -> Drag (Nm)/1
  DragFcn1/1 -> Saturation8/1
  ThrustFcn1/1 -> Saturation3/1
  Saturation4/1 -> Rotor Speed (r/s)/1, DragFcn1/1, ThrustFcn1/1
  RtrSpdFcn1/1 -> Saturation4/1

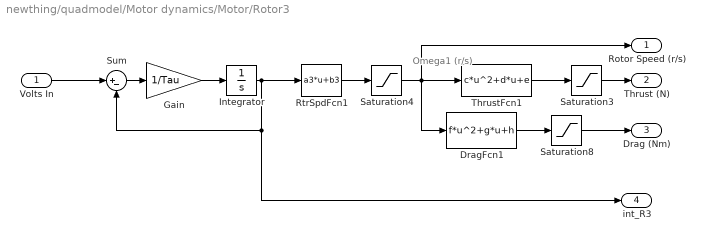
== system newthing/quadmodel/Motor dynamics/Motor/Rotor3 ==
  note: Omega1
      | (r/s)
  Volts In : Inport
  DragFcn1 : Fcn  Expr=f*u^2+g*u+h
  Gain : Gain  Gain=1/Tau
  Integrator : Integrator  InitialCondition=d_omega_R30
  RtrSpdFcn1 : Fcn  Expr=a3*u+b3
  Saturation3 : Saturate  UpperLimit=15  LowerLimit=0
  Saturation4 : Saturate  UpperLimit=250  LowerLimit=0
  Saturation8 : Saturate  UpperLimit=1  LowerLimit=0
  Sum : Sum  Inputs=|+-
  ThrustFcn1 : Fcn  Expr=c*u^2+d*u+e
  Rotor Speed (r/s) : Outport
  Thrust (N) : Outport  Port=2
  Drag (Nm) : Outport  Port=3
  int_R3 : Outport  Port=4
  wires:
  Volts In/1 -> Sum/1
  Sum/1 -> Gain/1
  Integrator/1 -> RtrSpdFcn1/1, int_R3/1, Sum/2
  Gain/1 -> Integrator/1
  Saturation3/1 -> Thrust (N)/1
  Saturation8/1 -> Drag (Nm)/1
  DragFcn1/1 -> Saturation8/1
  ThrustFcn1/1 -> Saturation3/1
  Saturation4/1 -> Rotor Speed (r/s)/1, DragFcn1/1, ThrustFcn1/1
  RtrSpdFcn1/1 -> Saturation4/1

== system newthing/quadmodel/Motor dynamics/Motor/Rotor4 ==
  note: Omega1
      | (r/s)
  Volts In : Inport
  DragFcn1 : Fcn  Expr=f*u^2+g*u+h
  Gain : Gain  Gain=1/Tau
  Integrator : Integrator  InitialCondition=d_omega_R40
  RtrSpdFcn1 : Fcn  Expr=a4*u+b4
  Saturation3 : Saturate  UpperLimit=15  LowerLimit=0
  Saturation4 : Saturate  UpperLimit=250  LowerLimit=0
  Saturation8 : Saturate  UpperLimit=1  LowerLimit=0
  Sum : Sum  Inputs=|+-
  ThrustFcn1 : Fcn  Expr=c*u^2+d*u+e
  Rotor Speed (r/s) : Outport
  Thrust (N) : Outport  Port=2
  Drag (Nm) : Outport  Port=3
  int_R4 : Outport  Port=4
  wires:
  Volts In/1 -> Sum/1
  Sum/1 -> Gain/1
  Integrator/1 -> RtrSpdFcn1/1, int_R4/1, Sum/2
  Gain/1 -> Integrator/1
  Saturation3/1 -> Thrust (N)/1
  Saturation8/1 -> Drag (Nm)/1
  DragFcn1/1 -> Saturation8/1
  ThrustFcn1/1 -> Saturation3/1
  Saturation4/1 -> Rotor Speed (r/s)/1, DragFcn1/1, ThrustFcn1/1
  RtrSpdFcn1/1 -> Saturation4/1

== matlab function KalmanFilter/Kalman Filter ==
  data: x_t_t input double; S_t_t input double; y_t1 input double; u_t input double; U1 input double; U2 input double; U3 input double; U4 input double; Omega input double; A input double; x_t1_t1 output double; B input double; C input double; G input double; H input double; Sv input double; Sw input double; S_t1_t1 output double; K output double; dt input double; ga input double; m input double; Ixx input double; Iyy input double; Izz input double; Jr input double; L input double
function [x_t1_t1,S_t1_t1,K] = fcn(x_t_t,S_t_t,y_t1,u_t,U1,U2,U3, ...
    U4,Omega,A,B,C,G,H,Sv,Sw,dt,ga,m,Ixx,Iyy,Izz,Jr,L)
%% This is a linear kalman filter! woooooo
    x_t1_t1 = zeros(16,1);
    S_t1_t1 = zeros(16,16);
    K = zeros(16,16);
    I = eye(16);
    x_t1_t = zeros(16,1);
    
    %nonlinear dynamics, linear for the rotor speed stuff
    x_t1_t(1) = x_t_t(2);
    x_t1_t(2) = (U1/m)*(cos(x_t_t(7))*sin(x_t_t(9))*cos(x_t_t(11)) ...
        + sin(x_t_t(7))*sin(x_t_t(11)));
    x_t1_t(3) = x_t_t(4);
    x_t1_t(4) = (U1/m)*(cos(x_t_t(7))*sin(x_t_t(9))*sin(x_t_t(11)) ...
        - sin(x_t_t(7))*cos(x_t_t(11)));
    x_t1_t(5) = x_t_t(6);
    x_t1_t(6) = -ga + (cos(x_t_t(7))*cos(x_t_t(9))*(U1/m));
    x_t1_t(7) = x_t_t(8);
    x_t1_t(8) = (x_t_t(12)*x_t_t(10)*((Iyy-Izz)/Ixx)) ...
        - (Jr/Ixx)*x_t_t(10)*Omega + (L/Ixx)*U2;
    x_t1_t(9) = x_t_t(10);
    x_t1_t(10) = (x_t_t(12)*x_t_t(8)*((Izz-Ixx)/Iyy)) ... 
        - (Jr/Iyy)*x_t_t(8)*Omega + (L/Iyy)*U3;
    x_t1_t(11) = x_t_t(12);
    x_t1_t(12) = (x_t_t(10)*x_t_t(8)*((Ixx-Iyy)/Izz)) - (L/Izz)*U4;
    x_t1_t(13:16) = A(13:16,13:16)*x_t_t(13:16) + B(13:16,:)*u_t;
    
    % prediction step
    x_t1_t= x_t1_t*dt + x_t_t;

    S_t1_t = (A*S_t_t*A.') + (G*Sw*G.');
    K = S_t1_t*((C.')*pinv((C*S_t1_t*C.')+(H*Sv*H.')));
    x_t1_t1 = x_t1_t + (K*(y_t1 - C*x_t1_t));
    S_t1_t1 = S_t1_t - K*C*(S_t1_t);   
    
    
    % predict
%     x_t1_t = (A*x_t_t + B*u_t)*dt + x_t_t;
%     S_t1_t = (A*S_t_t*A.') + Sw;
%     %update
%     y = y_t1 - C*x_t1_t;
%     S = Sv + C*S_t1_t*C.';
%     K = S_t1_t*(C.')*(pinv(S));
%     x_t1_t1 = x_t1_t + K*y;
%     S_t1_t1 = (I-K*C)*S_t1_t*((I-K*C).') + K*Sv*K.';
% deprecated
%     x_t1_t = A*x_t_t + B*u_t;
     

end
